simulink model "Pacemaker"  (R2023b)
settings: Solver=FixedStepAuto  StartTime=0.0  StopTime=inf  FixedStep=1e-3  RelTol=1e-3  EnableMultiTasking=on
undefined symbols (not defined in the file): D0, D1, D10, D11, D12, D13, D2, D3, D4, D5, D6, D7, D8, D9, PTA0, PTA1, PTA2, PTB23, PTB9, PTC16, PTC17, PTC2, PTC3, PTC4, PTD0, PTD1, PTD2, PTD3
libraries: frdmk64flib x18
settings Model: ExtModeTrigDuration=5  Creator=haley  LastModifiedBy=stivb
settings OptimizationCC: EnhancedBackFolding=on  PassReuseOutputArgsAs=Individual arguments  ZeroExternalMemoryAtStartup=off  ZeroInternalMemoryAtStartup=off  MaxStackSize=64  OptimizeBlockOrder=speed  DifferentSizesBufferReuse=on  OptimizationCustomize=off  EfficientTunableParamExpr=on
settings DebuggingCC: ParameterTunabilityLossMsg=error
settings HardwareCC: ProdBitPerPointer=32  ProdBitPerSizeT=32  ProdBitPerPtrDiffT=32  ProdLargestAtomicInteger=Long  ProdLargestAtomicFloat=Double  ProdWordSize=32  ProdHWDeviceType=ARM Compatible->ARM Cortex
settings SFSimCC: MATLABDynamicMemAlloc=off
settings RTWCC: Description=Embedded Coder  SystemTargetFile=ert.tlc  HardwareBoard=NXP FRDM-K64F  TLCOptions="-aInlineSetEventsForThisBaseRateFcn=TLC_FALSE -aSuppressMultiTaskScheduler=TLC_FALSE  -aRateBasedStepFcn=0"  TemplateMakefile=ert_default_tmf  Toolchain=GNU Tools for ARM Embedded Processors
settings CodeAppCC: ForceParamTrailComments=on  IgnoreCustomStorageClasses=off  OperatorAnnotations=on  SimulinkDataObjDesc=on  SFDataObjDesc=on  InsertBlockDesc=on
settings ERTTargetCC: ExtModeTransport=4  ExtModeMexFile=sendToCommService

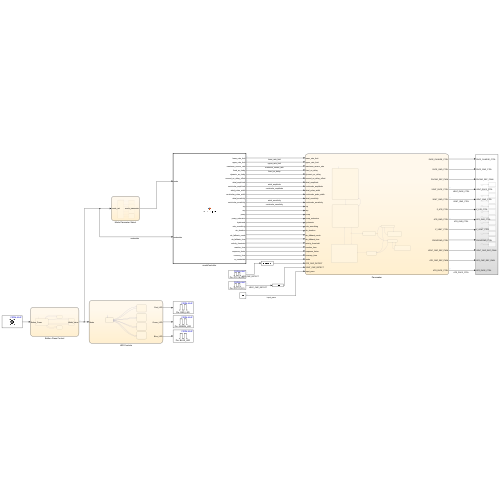
[thumbnail: Simulink's stored preview of the top-level diagram]
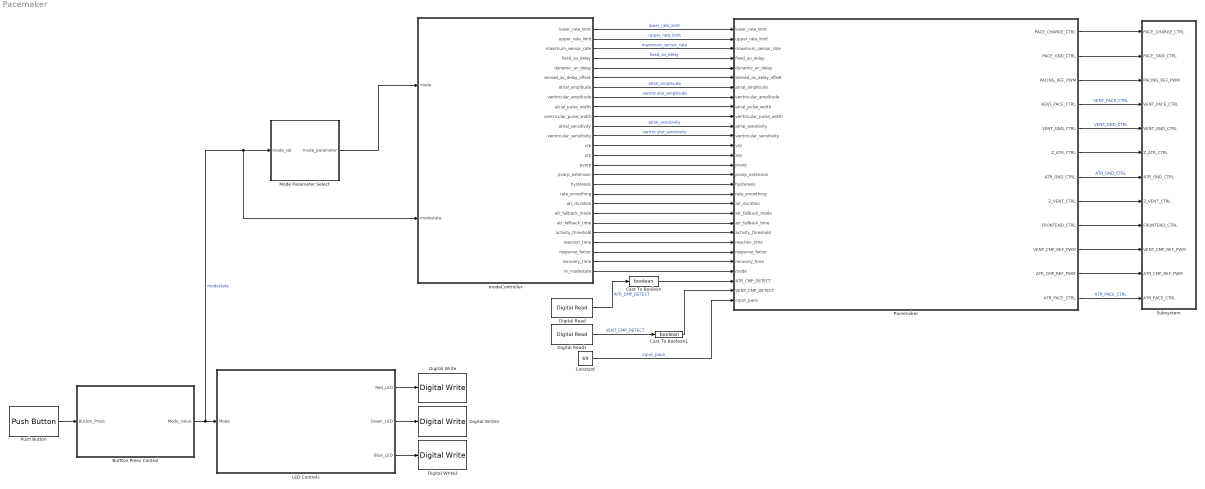
== system Pacemaker ==
  Buttton Press Control : Stateflow chart  TreatAsAtomicUnit=on
  Cast To Boolean : DataTypeConversion  OutDataTypeStr=boolean  SaturateOnIntegerOverflow=off  RndMeth=Floor
  Cast To Boolean1 : DataTypeConversion  OutDataTypeStr=boolean  SaturateOnIntegerOverflow=off  RndMeth=Floor
  Constant : Constant  Value=69
  Digital Read : frdmk64flib/Digital Read  Whichpin=PTC16 (D0)  SampleTime=-1
  Digital Read1 : frdmk64flib/Digital Read  Whichpin=PTC17 (D1)  SampleTime=-1
  Digital Write : frdmk64flib/Digital Write  Whichpin=RED_LED
  Digital Write1 : frdmk64flib/Digital Write  Whichpin=GREEN_LED
  Digital Write2 : frdmk64flib/Digital Write  Whichpin=BLUE_LED
  LED Controls : Stateflow chart  TreatAsAtomicUnit=on
  Mode Parameter Select : Stateflow chart  TreatAsAtomicUnit=on
  Pacemaker : Stateflow chart  TreatAsAtomicUnit=on
      settings: PortSchema="{\"entries\":[{\"content\":{\"sides\":[{\"content\":{\"connectorIds\":[\"In1\",\"In2\",\"In3\",\"In4\",\"In5\",\"In6\",\"In7\",\"In8\",\"In9\",\"In10\",\"In11\",\"In12\",\"In13\",\"In14\",\"In15\",\"In16\",\"In17\",\"In18\",\"In19\",\"In20\",\"In21\",\"In22\",\"In23\",\"In24\",\"In25\",\"In29\",\"In26\",\"In27\",\"In28\"]},\"type\":\"ConnectorPlacement.EquallySpacedRectSide\",\"uuid\":\"0d0b6505-f176-4343-a9b1-ea9b59cb1490\"},{\"content\":{\"connectorIds\":[\"Out3\",\"Out4\",\"Out5\",\"Out6\",\"Out7\",\"Out8\",\"Out2\",\"Out9\",\"Out10\",\"Out11\",\"Out12\",\"Out1\"],\"side\":\"RIGHT\"},\"type\":\"ConnectorPlacement.EquallySpacedRectSide\",\"uuid\":\"eab01ff7-bf59-4a22-8f26-311ca37acfb7\"},{\"content\":{\"side\":\"TOP\"},\"type\":\"ConnectorPlacement.EquallySpacedRectSide\",\"uuid\":\"e74717db-4bd0-436d-8de4-c78dd455d9ac\"}]},\"type\":\"ConnectorPlacement.EquallySpacedConnector\",\"uuid\":\"6be528cb-4290-4782-81af-91f8ed75056e\"}],\"packageUris\":[\"http://schema.mathworks.com/mf0/Connector/R2020b\"],\"version\":\"1.0\"}"
  Push Button : frdmk64flib/Push Button  Whichswitch=SW3  SampleTime1=-1
  Subsystem : Subsystem
  modeController : MATLAB Function  TreatAsAtomicUnit=on
  wires:
  LED Controls/3(Blue_LED) -> Digital Write2/1
  modeController/3(maximum_sensor_rate) -> Pacemaker/3(maximum_sensor_rate)  "maximum_sensor_rate"
  Push Button/1 -> Buttton Press Control/1(Button_Press)
  Pacemaker/3(PACE_CHARGE_CTRL) -> Subsystem/1(PACE_CHARGE_CTRL)
  Buttton Press Control/1(Mode_Value) -> modeController/2(modestate), Mode Parameter Select/1(mode_set), LED Controls/1(Mode)  "modestate"
  modeController/1(lower_rate_limit) -> Pacemaker/1(lower_rate_limit)  "lower_rate_limit"
  modeController/18(rate_smoothing) -> Pacemaker/18(rate_smoothing)
  LED Controls/1(Red_LED) -> Digital Write/1
  Pacemaker/5(PACING_REF_PWM) -> Subsystem/3(PACING_REF_PWM)
  LED Controls/2(Green_LED) -> Digital Write1/1
  modeController/2(upper_rate_limit) -> Pacemaker/2(upper_rate_limit)  "upper_rate_limit"
  modeController/4(fixed_av_delay) -> Pacemaker/4(fixed_av_delay)  "fixed_av_delay"
  Pacemaker/1(ATR_PACE_CTRL) -> Subsystem/12(ATR_PACE_CTRL)  "ATR_PACE_CTRL"
  modeController/5(dynamic_av_delay) -> Pacemaker/5(dynamic_av_delay)
  modeController/6(sensed_av_delay_offset) -> Pacemaker/6(sensed_av_delay_offset)
  modeController/7(atrial_amplitude) -> Pacemaker/7(atrial_amplitude)  "atrial_amplitude"
  Digital Read1/1 -> Cast To Boolean1/1  "VENT_CMP_DETECT"
  modeController/8(ventricular_amplitude) -> Pacemaker/8(ventricular_amplitude)  "ventricular_amplitude"
  Digital Read/1 -> Cast To Boolean/1  "ATR_CMP_DETECT"
  modeController/9(atrial_pulse_width) -> Pacemaker/9(atrial_pulse_width)
  modeController/16(pvarp_extension) -> Pacemaker/16(pvarp_extension)
  modeController/10(ventricular_pulse_width) -> Pacemaker/10(ventricular_pulse_width)
  modeController/21(atr_fallback_time) -> Pacemaker/21(atr_fallback_time)
  modeController/11(atrial_sensitivity) -> Pacemaker/11(atrial_sensitivity)  "atrial_sensitivity"
  modeController/24(response_factor) -> Pacemaker/24(response_factor)
  modeController/12(ventricular_sensitivity) -> Pacemaker/12(ventricular_sensitivity)  "ventricular_sensitivity"
  modeController/13(vrp) -> Pacemaker/13(vrp)
  modeController/14(arp) -> Pacemaker/14(arp)
  modeController/15(pvarp) -> Pacemaker/15(pvarp)
  modeController/17(hysteresis) -> Pacemaker/17(hysteresis)
  Pacemaker/8(Z_ATR_CTRL) -> Subsystem/6(Z_ATR_CTRL)
  modeController/19(atr_duration) -> Pacemaker/19(atr_duration)
  modeController/20(atr_fallback_mode) -> Pacemaker/20(atr_fallback_mode)
  modeController/22(activity_threshold) -> Pacemaker/22(activity_threshold)
  modeController/23(reaction_time) -> Pacemaker/23(reaction_time)
  modeController/25(recovery_time) -> Pacemaker/25(recovery_time)
  Constant/1 -> Pacemaker/28(input_pace)  "input_pace"
  Pacemaker/4(PACE_GND_CTRL) -> Subsystem/2(PACE_GND_CTRL)
  Pacemaker/6(VENT_PACE_CTRL) -> Subsystem/4(VENT_PACE_CTRL)  "VENT_PACE_CTRL"
  Pacemaker/7(VENT_GND_CTRL) -> Subsystem/5(VENT_GND_CTRL)  "VENT_GND_CTRL"
  Pacemaker/2(ATR_GND_CTRL) -> Subsystem/7(ATR_GND_CTRL)  "ATR_GND_CTRL"
  Pacemaker/9(Z_VENT_CTRL) -> Subsystem/8(Z_VENT_CTRL)
  Pacemaker/12(ATR_CMP_REF_PWM) -> Subsystem/11(ATR_CMP_REF_PWM)
  Pacemaker/10(FRONTEND_CTRL) -> Subsystem/9(FRONTEND_CTRL)
  Pacemaker/11(VENT_CMP_REF_PWM) -> Subsystem/10(VENT_CMP_REF_PWM)
  Mode Parameter Select/1(mode_parameter) -> modeController/1(mode)
  modeController/26(m_modestate) -> Pacemaker/29(mode)
  Cast To Boolean/1 -> Pacemaker/26(ATR_CMP_DETECT)
  Cast To Boolean1/1 -> Pacemaker/27(VENT_CMP_DETECT)

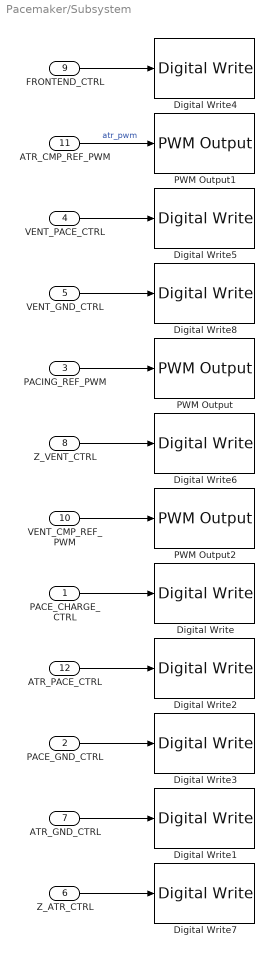
== system Pacemaker/Subsystem ==
  PACE_CHARGE_CTRL : Inport
  PACE_GND_CTRL : Inport  Port=2
  PACING_REF_PWM : Inport  Port=3
  VENT_PACE_CTRL : Inport  Port=4
  VENT_GND_CTRL : Inport  Port=5
  Z_ATR_CTRL : Inport  Port=6
  ATR_GND_CTRL : Inport  Port=7
  Z_VENT_CTRL : Inport  Port=8
  FRONTEND_CTRL : Inport  Port=9
  VENT_CMP_REF_PWM : Inport  Port=10
  ATR_CMP_REF_PWM : Inport  Port=11
  ATR_PACE_CTRL : Inport  Port=12
  Digital Write : frdmk64flib/Digital Write  Whichpin=PTB9 (D2)
  Digital Write1 : frdmk64flib/Digital Write  Whichpin=PTD2 (D11)
  Digital Write2 : frdmk64flib/Digital Write  Whichpin=PTA0 (D8)
  Digital Write3 : frdmk64flib/Digital Write  Whichpin=PTD0 (D10)
  Digital Write4 : frdmk64flib/Digital Write  Whichpin=PTD1 (D13)
  Digital Write5 : frdmk64flib/Digital Write  Whichpin=PTC4 (D9)
  Digital Write6 : frdmk64flib/Digital Write  Whichpin=PTC3 (D7)
  Digital Write7 : frdmk64flib/Digital Write  Whichpin=PTB23 (D4)
  Digital Write8 : frdmk64flib/Digital Write  Whichpin=PTD3 (D12)
  PWM Output : frdmk64flib/PWM Output  Whichpin=PTA2 (D5)  InitialFrequency=2000  InitialDutyCycle=0
  PWM Output1 : frdmk64flib/PWM Output  Whichpin=PTC2 (D6)  InitialFrequency=2000  InitialDutyCycle=0
  PWM Output2 : frdmk64flib/PWM Output  Whichpin=PTA1 (D3)  InitialFrequency=2000  InitialDutyCycle=0
  wires:
  VENT_PACE_CTRL/1 -> Digital Write5/1
  Z_VENT_CTRL/1 -> Digital Write6/1
  PACE_CHARGE_CTRL/1 -> Digital Write/1
  Z_ATR_CTRL/1 -> Digital Write7/1
  PACING_REF_PWM/1 -> PWM Output/1
  ATR_GND_CTRL/1 -> Digital Write1/1
  ATR_CMP_REF_PWM/1 -> PWM Output1/1  "atr_pwm"
  VENT_GND_CTRL/1 -> Digital Write8/1
  PACE_GND_CTRL/1 -> Digital Write3/1
  FRONTEND_CTRL/1 -> Digital Write4/1
  VENT_CMP_REF_PWM/1 -> PWM Output2/1
  ATR_PACE_CTRL/1 -> Digital Write2/1

== stateflow chart Pacemaker/Mode Parameter Select ==
  state OFF
    % Launch Point for determining mode, takes input
    % and selects proper functionality
    % if no mode selected (MODE 0), wait for it to change
  state AOO
    entry:
    %{
    Parameters Needed:
    LRL
    URL
    Atrial Amplitude
    Atrial Pulse Width
    %}
    mode_parameter = 0b1100001010000000000000000;
  state VOO
    entry:
    %{
    Parameters Needed:
    LRL
    URL
    Ventricular Amplitude
    Ventricular Pulse Width
    %}
    mode_parameter = 0b1100000101000000000000000;
  state AAI
    entry:
    %{
    Parameters Needed:
    Lower Rate Limit
    Upper Rate Limit
    Atrial Amplitude
    Atrial Pulse Width
    Hysteresis
    Rate Smoothing
    Atrial Sensitivity
    ARP
    PVARP
    %}
    mode_parameter = 0b1100001010100110110000000;
  state VVI
    entry:
    %{
    Parameters Needed:
    LRL
    URL
    Ventricle Amplitude
    Ventricle Pulse Width
    Hysteresis
    Rate Smoothing
    Ventricular Sensitivity
    VRP
    %}
    mode_parameter = 0b1100000101011000110000000;
  OFF -> OFF [order 1] : [mode_set == 0]
  OFF -> AOO [order 2] : [mode_set == 1]
  AOO -> OFF
  OFF -> VOO [order 3] : [mode_set == 2]
  VOO -> OFF
  OFF -> AAI [order 4] : [mode_set == 3]
  (default) -> OFF
  AAI -> OFF
  OFF -> VVI [order 5] : [mode_set == 4]
  VVI -> OFF
  data: mode_parameter output; mode_set input

== stateflow chart Pacemaker/Pacemaker ==
  state Initalize
    if atrial_amplitude >0
    atrial_pacing =1;
    ventricle_pacing =0;
    pwm_threshold = atrial_amplitude/5 * 100;
    atrial_sensing = 1;
    ventricular_sensing = 0;
    pulse_width = atrial_pulse_width;
    ATR_CMP_REF_PWM = atrial_sensitivity/3.3 * 100; %mV
    else
    ventricle_pacing =1;
    atrial_pacing = 0;
    pwm_threshold = ventricular_amplitude/5 * 100;
    atrial_sensing = 0;
    ventricular_sensing = 1;
    pulse_width = ventricular_pulse_width;
    VENT_CMP_REF_PWM = ventricular_sensitivity/3.3 * 100;
    end
    if input_pace >= lower_rate_limit && input_pace <= upper_rate_limit
    automatic_interval = double((1/input_pace)*60*1000); %msec
    elseif (input_pace < lower_rate_limit)
    automatic_interval = double((1/lower_rate_limit)*60*1000); %msec
    else
    automatic_interval = double((1/upper_rate_limit)*60*1000); %msec
    end
    if hysteresis
    escape_interval = double((1/hysteresis)*60*1000);
    else
    escape_interval = automatic_interval; %sanity check
    end
    if(atrial_sensitivity>0 || ventricular_sensitivity > 0)
    is_sensing = 1;
    else
    is_sensing = 0;
    end
    previous_mode = mode;
  state ChangeMode
  state Charge_C22_Discharge_C21
    entry:
    %Charge C22
    ATR_PACE_CTRL = 0;
    VENT_PACE_CTRL = 0;
    PACE_CHARGE_CTRL = 1;
    PACING_REF_PWM = pwm_threshold; %percentage
    %Discharge C21
    PACE_GND_CTRL = 1;
    VENT_PACE_CTRL = 0;
    Z_ATR_CTRL = 0;
    Z_VENT_CTRL = 0;
    ATR_PACE_CTRL = 0;
    ATR_GND_CTRL = atrial_pacing;
    VENT_GND_CTRL= ventricle_pacing;
  note: Mode has changed, go back to initialization state
  note: Atrial Sensing System
  state AtrialEventDetected
    entry:
    sensing_interval = escape_interval - double(arp);
  state AtrialSensing
  note: Set sensing interval to the escape interval since we are
      | using hysteresis pacing
  note: Enter sensing state
  state EnterSensing
    entry:
    FRONTEND_CTRL = true;
    sensing_interval = automatic_interval;
  note: Ventricle Sensing System
  state VentricularEventDetected
    entry:
    sensing_interval = escape_interval - double(vrp);
  state VentricularSensing
  note: If not in sensing, continue pacing at automatic interval
  state ChargeC21_and_DischargeC22
    %Creates the leading edge and sends pulse for X amount of time
    entry:
    PACE_CHARGE_CTRL = 0;
    PACE_GND_CTRL = 1;
    ATR_PACE_CTRL = atrial_pacing;
    ATR_GND_CTRL = 0;
    Z_ATR_CTRL = 0;
    Z_VENT_CTRL = 0;
    VENT_GND_CTRL = 0;
    VENT_PACE_CTRL = ventricle_pacing;
    %Recharge pulse is the current in the opposite direction due to C21
  state ExitSensing
    entry:
    FRONTEND_CTRL = false;
  note: No pulses detected within specified interval, exit sensing to return to pacing
  (default) -> Initalize
  ChangeMode -> Initalize : [after(20, msec)]
  VentricularSensing -> ChangeMode [order 3] : [hasChangedFrom(mode, previous_mode)]
  AtrialSensing -> ChangeMode [order 3] : [hasChangedFrom(mode, previous_mode)]
  Charge_C22_Discharge_C21 -> ChangeMode [order 1] : [hasChangedFrom(mode, previous_mode)]
  Initalize -> Charge_C22_Discharge_C21
  AtrialSensing -> AtrialEventDetected [order 1] : [hasChangedTo(ATR_CMP_DETECT, true)]
  (junction 100) -> AtrialSensing [order 1] : [atrial_sensing == 1 && after(arp, msec)]
  AtrialSensing -> ExitSensing [order 2] : [after(sensing_interval, msec)]
  AtrialEventDetected -> AtrialSensing : [after(arp, msec)]
  ChargeC21_and_DischargeC22 -> Charge_C22_Discharge_C21 : after(pulse_width, msec)
  Charge_C22_Discharge_C21 -> (junction 106) [order 2]
  EnterSensing -> (junction 100)
  (junction 106) -> EnterSensing [order 2] : [is_sensing == 1]
  (junction 100) -> VentricularSensing [order 2] : [ventricular_sensing == 1 && after(vrp, msec)]
  (junction 106) -> ChargeC21_and_DischargeC22 [order 1] : [is_sensing == 0 && after(automatic_interval, msec)]
  VentricularSensing -> VentricularEventDetected [order 1] : [hasChangedTo(VENT_CMP_DETECT, true)]
  VentricularSensing -> ExitSensing [order 2] : [after(sensing_interval, msec)]
  VentricularEventDetected -> VentricularSensing : [after(vrp, msec)]
  ExitSensing -> ChargeC21_and_DischargeC22
  data: ATR_PACE_CTRL output; ATR_GND_CTRL output; PACE_CHARGE_CTRL output; PACE_GND_CTRL output; PACING_REF_PWM output; VENT_PACE_CTRL output; VENT_GND_CTRL output; Z_ATR_CTRL output; Z_VENT_CTRL output; lower_rate_limit input; upper_rate_limit input; maximum_sensor_rate input; fixed_av_delay input; dynamic_av_delay input; sensed_av_delay_offset input; atrial_amplitude input; ventricular_amplitude input; atrial_pulse_width input; ventricular_pulse_width input; atrial_sensitivity input; ventricular_sensitivity input; vrp input; arp input; pvarp input; pvarp_extension input; hysteresis input; rate_smoothing input; atr_duration input; atr_fallback_mode input; atr_fallback_time input; activity_threshold input; reaction_time input; response_factor input; recovery_time input; FRONTEND_CTRL output boolean; ATR_CMP_DETECT input boolean; VENT_CMP_DETECT input boolean; sensing_interval local; atrial_pacing local; pulse_width local; pwm_threshold local; ventricle_pacing local; ventricular_sensing local; atrial_sensing local; VENT_CMP_REF_PWM output; ATR_CMP_REF_PWM output; automatic_interval local; escape_interval local; input_pace input; is_sensing local; mode input; previous_mode local

== stateflow chart Pacemaker/LED Controls ==
  state AOO
    entry:
    Red_LED = 1
    Green_LED = 0
    Blue_LED = 0
  state VOO
    entry:
    Red_LED = 0
    Green_LED = 1
    Blue_LED = 0
  state Controller
  state AAI
    entry:
    Red_LED = 0
    Green_LED = 0
    Blue_LED = 1
  state VVI
    entry:
    Red_LED = 1
    Green_LED = 0
    Blue_LED = 1
  Controller -> AOO [order 1] : [Mode == 1]
  AOO -> Controller
  (default) -> Controller
  Controller -> VOO [order 2] : [Mode == 2]
  VOO -> Controller
  Controller -> AAI [order 3] : [Mode == 3]
  AAI -> Controller
  Controller -> VVI [order 4] : [Mode == 4]
  VVI -> Controller
  data: Mode input; Red_LED output; Green_LED output; Blue_LED output

== stateflow chart Pacemaker/Buttton Press Control ==
  state AOO
    entry:
    Mode_Value = 1
  state VOO
    entry:
    Mode_Value = 2
  state Controller
    entry:
    counter = 1 + mod(counter,4) %mod  4
  state AAI
    entry:
    Mode_Value = 3
  state VVI
    entry:
    Mode_Value = 4
  AOO -> Controller : [Button_Press == 0]
  Controller -> AOO [order 1] : [Button_Press == 1 && counter == 1]
  (default) -> Controller
  Controller -> VOO [order 2] : [Button_Press  == 1 && counter == 2]
  VOO -> Controller : [Button_Press  == 0]
  Controller -> AAI [order 3] : [Button_Press  == 1 && counter == 3]
  AAI -> Controller : [Button_Press  == 0]
  VVI -> Controller : [Button_Press  == 0]
  Controller -> VVI [order 4] : [Button_Press  == 1 && counter == 4]
  data: Mode_Value output; Button_Press input; counter local =0

== matlab function Pacemaker/modeController ==
  data: mode input; lower_rate_limit output; upper_rate_limit output; maximum_sensor_rate output; fixed_av_delay output; dynamic_av_delay output; sensed_av_delay_offset output; atrial_amplitude output; ventricular_amplitude output; atrial_pulse_width output; ventricular_pulse_width output; atrial_sensitivity output; ventricular_sensitivity output; vrp output; arp output; pvarp output; pvarp_extension output; hysteresis output; rate_smoothing output; atr_duration output; atr_fallback_mode output; atr_fallback_time output; activity_threshold output; reaction_time output; response_factor output; recovery_time output; m_modestate output; modestate input



function [lower_rate_limit, upper_rate_limit, maximum_sensor_rate, fixed_av_delay, dynamic_av_delay, sensed_av_delay_offset, atrial_amplitude, ventricular_amplitude, atrial_pulse_width, ventricular_pulse_width, atrial_sensitivity, ventricular_sensitivity, vrp, arp, pvarp, pvarp_extension, hysteresis, rate_smoothing, atr_duration, atr_fallback_mode, atr_fallback_time, activity_threshold, reaction_time, response_factor, recovery_time, m_modestate] = modeAdapter(mode, modestate)
    
    
    % Start by taking the mode input as a binary number, and extrapolating
    % all the active parameters.
    % Should return 1 if true and 0 if false
    %mode_vector = num2str(mode) - '0'; %convert the input to a list
    %N = 1994;
    
    lower_rate_limit = bitand(mode, 0b1000000000000000000000000); %Parameter 1
    upper_rate_limit = bitand(mode, 0b0100000000000000000000000); %Parameter 2
    maximum_sensor_rate = bitand(mode, 0b0010000000000000000000000); %Parameter 3
    fixed_av_delay = bitand(mode, 0b0001000000000000000000000); %Parameter 4
    dynamic_av_delay = bitand(mode, 0b0000100000000000000000000); %Parameter 5
    sensed_av_delay_offset = bitand(mode, 0b0000010000000000000000000); %Parameter 6
    atrial_amplitude = bitand(mode, 0b0000001000000000000000000); %Parameter 7
    ventricular_amplitude = bitand(mode, 0b0000000100000000000000000); %Parameter 8
    atrial_pulse_width = bitand(mode, 0b0000000010000000000000000); %Parameter 9
    ventricular_pulse_width = bitand(mode, 0b0000000001000000000000000); %Parameter 10
    atrial_sensitivity = bitand(mode, 0b0000000000100000000000000); %Parameter 11
    ventricular_sensitivity = bitand(mode, 0b0000000000010000000000000); %Parameter 12
    vrp = bitand(mode, 0b0000000000001000000000000); %Parameter 13
    arp = bitand(mode, 0b0000000000000100000000000); %Parameter 14
    pvarp = bitand(mode, 0b0000000000000010000000000); %Parameter 15
    pvarp_extension = bitand(mode, 0b0000000000000001000000000); %Parameter 16
    hysteresis = bitand(mode, 0b0000000000000000100000000); %Parameter 17
    rate_smoothing = bitand(mode, 0b0000000000000000010000000); %Parameter 18
    atr_duration = bitand(mode, 0b0000000000000000001000000); %Parameter 19
    atr_fallback_mode = bitand(mode, 0b0000000000000000000100000); %Parameter 20
    atr_fallback_time = bitand(mode, 0b0000000000000000000010000); %Parameter 21
    activity_threshold = bitand(mode, 0b0000000000000000000001000); %Parameter 22
    reaction_time = bitand(mode, 0b0000000000000000000000100); %Parameter 23
    response_factor = bitand(mode, 0b0000000000000000000000010); %Parameter 24
    recovery_time = bitand(mode, 0b0000000000000000000000001); %Parameter 25
    m_modestate = modestate;

    set_lower_rate_limit = (40); %Parameter 1
    set_upper_rate_limit = (100); %Parameter 2
    set_maximum_sensor_rate = (100); %Parameter 3
    set_fixed_av_delay = (100); %Parameter 4
    set_dynamic_av_delay = (1); %Parameter 5
    set_sensed_av_delay_offset = (-50); %Parameter 6
    set_atrial_amplitude = (4); %Parameter 7
    set_ventricular_amplitude = (4); %Parameter 8
    set_atrial_pulse_width = (5); %Parameter 9
    set_ventricular_pulse_width = (5); %Parameter 10
    set_atrial_sensitivity = (0.75); %Parameter 11
    set_ventricular_sensitivity = (2.5); %Parameter 12
    set_vrp = (300); %Parameter 13
    set_arp = (300); %Parameter 14
    set_pvarp = (300); %Parameter 15
    set_pvarp_extension = (200); %Parameter 16
    set_hysteresis = (set_lower_rate_limit); %Parameter 17
    set_rate_smoothing = (15); %Parameter 18
    set_atr_duration = (10); %Parameter 19
    set_atr_fallback_mode = (1); %Parameter 20
    set_atr_fallback_time = (3); %Parameter 21
    set_activity_threshold = (3); %Parameter 22
    set_reaction_time = (30); %Parameter 23
    set_response_factor = (10); %Parameter 24
    set_recovery_time = (10); %Parameter 25
    
    length = 25;
    
    input_list = [lower_rate_limit, upper_rate_limit, maximum_sensor_rate, fixed_av_delay, dynamic_av_delay, sensed_av_delay_offset, atrial_amplitude, ventricular_amplitude, atrial_pulse_width, ventricular_pulse_width, atrial_sensitivity, ventricular_sensitivity, vrp, arp, pvarp, pvarp_extension, hysteresis, rate_smoothing, atr_duration, atr_fallback_mode, atr_fallback_time, activity_threshold, reaction_time, response_factor, recovery_time];
    parameter_list = [set_lower_rate_limit, set_upper_rate_limit, set_maximum_sensor_rate, set_fixed_av_delay, set_dynamic_av_delay, set_sensed_av_delay_offset, set_atrial_amplitude, set_ventricular_amplitude, set_atrial_pulse_width, set_ventricular_pulse_width, set_atrial_sensitivity, set_ventricular_sensitivity, set_vrp, set_arp, set_pvarp, set_pvarp_extension, set_hysteresis, set_rate_smoothing, set_atr_duration, set_atr_fallback_mode, set_atr_fallback_time, set_activity_threshold, set_reaction_time, set_response_factor, set_recovery_time];
    
    for i = 1:length
        if input_list(i) ~= 0
            input_list(i) = parameter_list(i);
        end
    end
    
    %Redeclare the values
    lower_rate_limit = input_list(1); %Parameter 1
    upper_rate_limit = input_list(2); %Parameter 2
    maximum_sensor_rate = input_list(3); %Parameter 3
    fixed_av_delay = input_list(4); %Parameter 4
    dynamic_av_delay = input_list(5); %Parameter 5
    sensed_av_delay_offset = input_list(6); %Parameter 6
    atrial_amplitude = input_list(7); %Parameter 7
    ventricular_amplitude = input_list(8); %Parameter 8
    atrial_pulse_width = input_list(9); %Parameter 9
    ventricular_pulse_width = input_list(10); %Parameter 10
    atrial_sensitivity = input_list(11); %Parameter 11
    ventricular_sensitivity = input_list(12); %Parameter 12
    vrp = input_list(13); %Parameter 13
    arp = input_list(14); %Parameter 14
    pvarp = input_list(15); %Parameter 15
    pvarp_extension = input_list(16); %Parameter 16
    hysteresis = input_list(17); %Parameter 17
    rate_smoothing = input_list(18); %Parameter 18
    atr_duration = input_list(19); %Parameter 19
    atr_fallback_mode = input_list(20); %Parameter 20
    atr_fallback_time = input_list(21); %Parameter 21
    activity_threshold = input_list(22); %Parameter 22
    reaction_time = input_list(23); %Parameter 23
    response_factor = input_list(24); %Parameter 24
    recovery_time = input_list(25); %Parameter 25
    
    
end
